simulink model "integrateFireNeuron"  (Simulink 7.6)
settings: Solver=ode45  StartTime=0.0  StopTime=5  FixedStep=0.0005  RelTol=1e-3
libraries: simulink x2
settings Model: Creator=sstavisk  LastModifiedBy=sstavisk
settings SolverCC: ShapePreserveControl=EnableAll

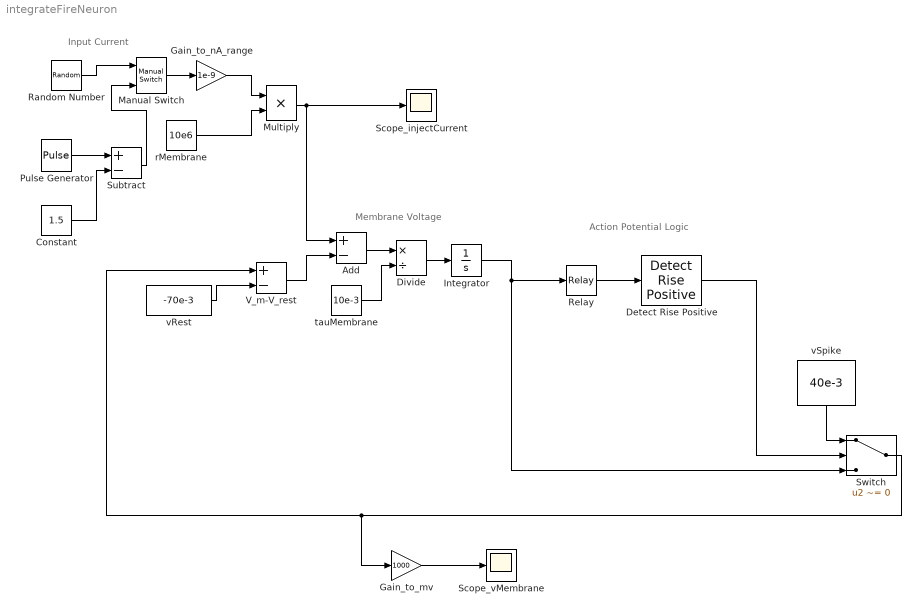
== system integrateFireNeuron ==
  note: Input Current
  note: Membrane Voltage
  note: Action Potential Logic
  Add : Sum  Inputs=+-
  Constant : Constant  Value=1.5
  Detect Rise Positive : simulink/Logic and Bit Operations/Detect Rise Positive  SystemSampleTime=-1  vinit=0
  Divide : Product  Inputs=*/  RndMeth=Zero
  Gain_to_mv : Gain  Gain=1000
  Gain_to_nA_range : Gain  Gain=1e-9
  Integrator : Integrator  InitialCondition=-70e-3  ContinuousStateAttributes='vMembrane'
  Manual Switch : simulink/Signal Routing/Manual Switch  SystemSampleTime=-1  sw=1  action=0  varsize=off
  Multiply : Product  Inputs=**  RndMeth=Zero
  Pulse Generator : DiscretePulseGenerator  PulseType=Time based  Amplitude=3  Period=.100  PulseWidth=50
  Random Number : RandomNumber  Seed=1  SampleTime=0.05  VectorParams1D=off
  Relay : Relay  OnSwitchValue=-55e-3  OffSwitchValue=-60e-3
  Scope_injectCurrent : Scope
      settings: TimeRange=5  YMin=-0.04  YMax=0.03000000000000001
  Scope_vMembrane : Scope
      settings: TimeRange=5  YMin=-100  YMax=50
  Subtract : Sum  Inputs=+-
  Switch : Switch  Criteria=u2 ~= 0
  V_m-V_rest : Sum  Inputs=+-
  rMembrane : Constant  Value=10e6
  tauMembrane : Constant  Value=10e-3
  vRest : Constant  Value=-70e-3
  vSpike : Constant  Value=40e-3
  wires:
  Integrator/1 -> Switch/3, Relay/1
  Add/1 -> Divide/1
  tauMembrane/1 -> Divide/2
  vRest/1 -> V_m-V_rest/2
  V_m-V_rest/1 -> Add/2
  rMembrane/1 -> Multiply/2
  Gain_to_mv/1 -> Scope_vMembrane/1
  Multiply/1 -> Scope_injectCurrent/1, Add/1
  Gain_to_nA_range/1 -> Multiply/1
  Relay/1 -> Detect Rise Positive/1
  vSpike/1 -> Switch/1
  Switch/1 -> V_m-V_rest/1, Gain_to_mv/1
  Divide/1 -> Integrator/1
  Detect Rise Positive/1 -> Switch/2
  Manual Switch/1 -> Gain_to_nA_range/1
  Random Number/1 -> Manual Switch/1
  Pulse Generator/1 -> Subtract/1
  Constant/1 -> Subtract/2
  Subtract/1 -> Manual Switch/2
